simulink model "MBE_Simulation_04_Template_14_11_final"  (R2017b)
settings: Solver=FixedStepAuto  StartTime=0.0  StopTime=inf  FixedStep=0.05  RelTol=1e-3
libraries: simulink x67, canmsglib x4, instrumentlib x2, realtime_pacer_lib x1, hdlsllib x1
(part 1 of 4)
settings Model: Creator=holtv  LastModifiedBy=labadmin
settings CodeAppCC: StateflowObjectComments=on

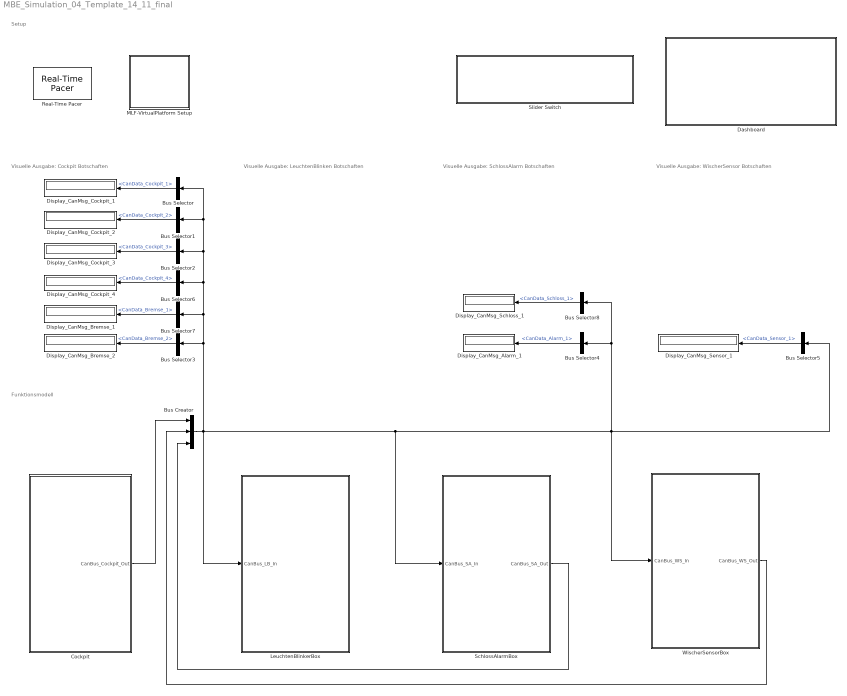
== system MBE_Simulation_04_Template_14_11_final ==
  note: Setup
  note: Visuelle Ausgabe: Cockpit Botschaften
  note: Funktionsmodell
  note: Visuelle Ausgabe: SchlossAlarm Botschaften
  note: Visuelle Ausgabe: LeuchtenBlinken Botschaften
  note: Visuelle Ausgabe: WischerSensor Botschaften
  Bus Creator : BusCreator  Inputs=3
  Bus Selector : BusSelector  OutputSignals=CanBus_Cockpit.CanMsg_Cockpit_1.CanData_Cockpit_1
  Bus Selector1 : BusSelector  OutputSignals=CanBus_Cockpit.CanMsg_Cockpit_2.CanData_Cockpit_2
  Bus Selector2 : BusSelector  OutputSignals=CanBus_Cockpit.CanMsg_Cockpit_3.CanData_Cockpit_3
  Bus Selector3 : BusSelector  OutputSignals=CanBus_Cockpit.CanMsg_Bremse_2.CanData_Bremse_2
  Bus Selector4 : BusSelector  OutputSignals=CanBus_SA.CanMsg_Alarm_1.CanData_Alarm_1
  Bus Selector5 : BusSelector  OutputSignals=CanBus_WS.CanMsg_Sensor_1.CanData_Sensor_1
  Bus Selector6 : BusSelector  OutputSignals=CanBus_Cockpit.CanMsg_Cockpit_4.CanData_Cockpit_4
  Bus Selector7 : BusSelector  OutputSignals=CanBus_Cockpit.CanMsg_Bremse_1.CanData_Bremse_1
  Bus Selector8 : BusSelector  OutputSignals=CanBus_SA.CanMsg_Schloss_1.CanData_Schloss_1
  Cockpit : Subsystem
  Dashboard : Subsystem
      mask Display: image('resources/simulink-dashboard.png');
  Display_CanMsg_Alarm_1 : Display
      settings: Format=binary (Stored Integer)
  Display_CanMsg_Bremse_1 : Display
      settings: Format=binary (Stored Integer)
  Display_CanMsg_Bremse_2 : Display
      settings: Format=binary (Stored Integer)
  Display_CanMsg_Cockpit_{1..4} (4 alike) : Display
      settings: Format=binary (Stored Integer)
  Display_CanMsg_Schloss_1 : Display
      settings: Format=binary (Stored Integer)
  Display_CanMsg_Sensor_1 : Display
      settings: Format=binary (Stored Integer)
  LeuchtenBlinkerBox : Subsystem
  MLF-VirtualPlatform Setup : Subsystem
  Real-Time Pacer : realtime_pacer_lib/Real-Time Pacer  simTimePerRealTime=1
  SchlossAlarmBox : Subsystem
  Slider Switch : Subsystem  DialogController=hmiCreateDDGDialog  IsWebBlock=on  mask(MWDashboardBlock){webBlockId=66e1d68e-5f4b-49dc-992d-d286b9288448, webBlockType=sliderswitch, ShowInLibBrowser=on, ShowInitialText=on, HMISrcModelName=MBE_Simulation_04_Template_14_11_final}
      mask prompts: webBlockId "WebBlock Id"; webBlockType "WebBlock Type"; HMISrcModelName "Source Model"
      mask help: Set on/off value to tune parameters or variables.
      mask Help: helpview([docroot '/mapfiles/simulink.map'], 'hmi_switch')
      mask Display:
      | if strcmp(get_param(bdroot(gcb),'BlockDiagramType'),'library')
      |  image([(matlabroot) '/toolbox/simulink/hmi/icons/SliderSwitch.png'])
      | end
  WischerSensorBox : Subsystem
  wires:
  Bus Creator/1 -> Bus Selector/1, Bus Selector1/1, Bus Selector2/1, Bus Selector6/1, Bus Selector7/1, Bus Selector3/1, Bus Selector5/1, Bus Selector8/1, Bus Selector4/1, WischerSensorBox/1(CanBus_WS_In), SchlossAlarmBox/1(CanBus_SA_In), LeuchtenBlinkerBox/1(CanBus_LB_In)
  Bus Selector/1 -> Display_CanMsg_Cockpit_1/1  "<CanData_Cockpit_1>"
  Bus Selector1/1 -> Display_CanMsg_Cockpit_2/1  "<CanData_Cockpit_2>"
  Bus Selector2/1 -> Display_CanMsg_Cockpit_3/1  "<CanData_Cockpit_3>"
  Bus Selector3/1 -> Display_CanMsg_Bremse_2/1  "<CanData_Bremse_2>"
  Bus Selector4/1 -> Display_CanMsg_Alarm_1/1  "<CanData_Alarm_1>"
  Bus Selector5/1 -> Display_CanMsg_Sensor_1/1  "<CanData_Sensor_1>"
  Cockpit/1(CanBus_Cockpit_Out) -> Bus Creator/1
  Bus Selector6/1 -> Display_CanMsg_Cockpit_4/1  "<CanData_Cockpit_4>"
  Bus Selector7/1 -> Display_CanMsg_Bremse_1/1  "<CanData_Bremse_1>"
  Bus Selector8/1 -> Display_CanMsg_Schloss_1/1  "<CanData_Schloss_1>"
  SchlossAlarmBox/1(CanBus_SA_Out) -> Bus Creator/3
  WischerSensorBox/1(CanBus_WS_Out) -> Bus Creator/2

== system MBE_Simulation_04_Template_14_11_final/Cockpit ==
  note: Applikation
  note: Simulation
  CanBus_Cockpit : Subsystem
  CanCoder_Bremse_1 : Subsystem
  CanCoder_Bremse_2 : Subsystem
  CanCoder_Cockpit_1 : Subsystem
  CanCoder_Cockpit_2 : Subsystem
  CanCoder_Cockpit_3 : Subsystem
  CanCoder_Cockpit_4 : Subsystem
  CanTransmit_Bremse_1 : Subsystem
  CanTransmit_Bremse_2 : Subsystem
  CanTransmit_Cockpit_1 : Subsystem
  CanTransmit_Cockpit_2 : Subsystem
  CanTransmit_Cockpit_3 : Subsystem
  CanTransmit_Cockpit_4 : Subsystem
  PanelInput_Cockpit : Subsystem
  CanBus_Cockpit_Out : Outport
  wires:
  PanelInput_Cockpit/1(LichtSwitch_Out) -> CanCoder_Cockpit_1/1(Lichtschalter_In)
  PanelInput_Cockpit/2(BlinkerSwitch_Out) -> CanCoder_Cockpit_1/2(Blinkerhebel_In)
  PanelInput_Cockpit/3(WarnblinkerSwitch_Out) -> CanCoder_Cockpit_1/3(Warnblinker)
  PanelInput_Cockpit/4(WischerSwitch_Out) -> CanCoder_Cockpit_2/1(WischerSwitch_In)
  PanelInput_Cockpit/5(WischWaschButton_Out) -> CanCoder_Cockpit_2/2(WischWaschButton_In)
  PanelInput_Cockpit/6(ScheibenheizungSwitch_Out) -> CanCoder_Cockpit_2/3(ScheibenheizungSwitch_In)
  PanelInput_Cockpit/7(TemperaturSlider_Out) -> CanCoder_Cockpit_2/4(TemperaturSlider_In)
  PanelInput_Cockpit/8(AlarmResetButton_Out) -> CanCoder_Cockpit_3/1(AlarmResetButton_In)
  PanelInput_Cockpit/13(GeschwindigkeitsSlider_Out) -> CanCoder_Bremse_2/1(GeschwindigkeitsSlider_In)
  PanelInput_Cockpit/9(IgnitionSwitch_Out) -> CanCoder_Cockpit_4/1(IgnitionSwitch_In)
  PanelInput_Cockpit/10(BremseButton_Out) -> CanCoder_Bremse_1/1(Bremse_In)
  PanelInput_Cockpit/11(WarnbremsungButton_Out) -> CanCoder_Bremse_1/2(Warnbremsung_In)
  PanelInput_Cockpit/12(NotbremsungButton_Out) -> CanCoder_Bremse_1/3(Notbremsungl_In)
  CanCoder_Cockpit_1/1(CanData_Cockpit_1) -> CanTransmit_Cockpit_1/1(CanData_Cockpit_1_In)  "CanData_Cockpit_1"
  CanCoder_Cockpit_1/2(CanTrigger_Cockpit_1) -> CanTransmit_Cockpit_1/2(CanTrigger_Cockpit_1_In)  "CanTrigger_Cockpit_1"
  CanCoder_Cockpit_2/1(CanData_Cockpit_2) -> CanTransmit_Cockpit_2/1(CanData_Cockpit_2_In)  "CanData_Cockpit_2"
  CanCoder_Cockpit_2/2(CanTrigger_Cockpit_2) -> CanTransmit_Cockpit_2/2(CanTrigger_Cockpit_2_In)  "CanTrigger_Cockpit_2"
  CanCoder_Cockpit_3/1(CanData_Cockpit_3) -> CanTransmit_Cockpit_3/1(CanData_Cockpit_3_In)  "CanData_Cockpit_3"
  CanCoder_Cockpit_3/2(CanTrigger_Cockpit_3) -> CanTransmit_Cockpit_3/2(CanTrigger_Cockpit_3_In)  "CanTrigger_Cockpit_3"
  CanCoder_Cockpit_4/1(CanData_Cockpit_4) -> CanTransmit_Cockpit_4/1(CanData_Cockpit_4_In)  "CanData_Cockpit_4"
  CanCoder_Cockpit_4/2(CanTrigger_Cockpit_4) -> CanTransmit_Cockpit_4/2(CanTrigger_Cockpit_4_In)  "CanTrigger_Cockpit_4"
  CanCoder_Bremse_1/1(CanData_Bremse_1) -> CanTransmit_Bremse_1/1(CanData_Bremse_1_In)  "CanData_Bremse_1"
  CanCoder_Bremse_1/2(CanTrigger_Bremse_1) -> CanTransmit_Bremse_1/2(CanTrigger_Bremse_1_In)  "CanTrigger_Bremse_1"
  CanCoder_Bremse_2/1(CanMsg_Bremse_2) -> CanTransmit_Bremse_2/1(CanData_Bremse_2_In)  "CanData_Bremse_2"
  CanCoder_Bremse_2/2(CanTrigger_Bremse_2) -> CanTransmit_Bremse_2/2(CanTrigger_Bremse_2_In)  "CanTrigger_Bremse_2"
  CanTransmit_Cockpit_1/1(CanMsg_Cockpit_1_Out) -> CanBus_Cockpit/1("CanMsg_Cockpit_1_In ")  "CanMsg_Cockpit_1"
  CanTransmit_Cockpit_2/1(CanMsg_Cockpit_2_Out) -> CanBus_Cockpit/2(CanMsg_Cockpit_2_In)  "CanMsg_Cockpit_2"
  CanTransmit_Cockpit_3/1(CanMsg_Cockpit_3_Out) -> CanBus_Cockpit/3(CanMsg_Cockpit_3_In)  "CanMsg_Cockpit_3"
  CanTransmit_Cockpit_4/1(CanMsg_Cockpit_4_Out) -> CanBus_Cockpit/4(CanMsg_Cockpit_4_In)  "CanMsg_Cockpit_4"
  CanTransmit_Bremse_1/1(CanTrigger_Bremse_1_Out) -> CanBus_Cockpit/5(CanMsg_Bremse_1_In)  "CanMsg_Bremse_1"
  CanTransmit_Bremse_2/1(CanMsg_Bremse_2_Out) -> CanBus_Cockpit/6(CanMsg_Bremse_2_In)  "CanMsg_Bremse_2"
  CanBus_Cockpit/1(CanBus_Cockpit_Out) -> CanBus_Cockpit_Out/1  "CanBus_Cockpit"

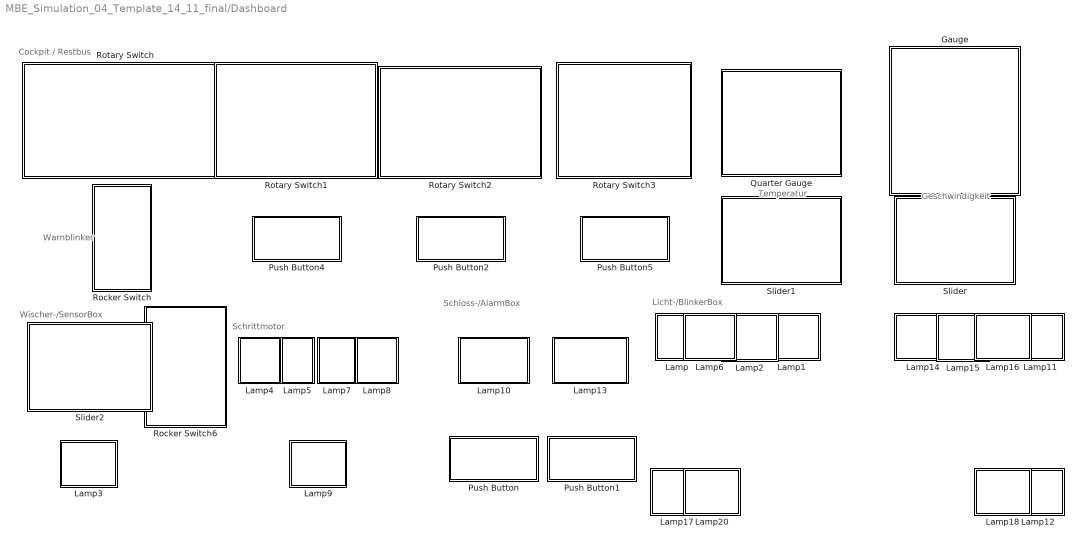
== system MBE_Simulation_04_Template_14_11_final/Dashboard ==
  note: Temperatur
  note: Geschwindigkeit
  note: Warnblinker
  note: Schloss-/AlarmBox
  note: Schrittmotor
  note: Wischer-/SensorBox
  note: Cockpit / Restbus
  note: Licht-/BlinkerBox
  Gauge : Subsystem  DialogController=hmiCreateDDGDialog  IsWebBlock=on  mask(MWDashboardBlock){webBlockId=ca009e5b-bc53-4e09-90f4-318b3a316375, webBlockType=circulargauge, ShowInLibBrowser=on, ShowInitialText=on, HMISrcModelName=MBE_Simulation_04_Template_14_11_final}
      mask prompts: webBlockId "WebBlock Id"; webBlockType "WebBlock Type"; HMISrcModelName "Source Model"
      mask help: Display an input value on a circular scale.
      mask Help: helpview([docroot '/mapfiles/simulink.map'], 'hmi_gauge')
      mask Display:
      | if strcmp(get_param(bdroot(gcb),'BlockDiagramType'),'library')
      |  image([(matlabroot) '/toolbox/simulink/hmi/icons/CircularGauge.png'])
      | end
  Lamp : Subsystem  DialogController=hmiCreateDDGDialog  IsWebBlock=on  mask(MWDashboardBlock){webBlockId=81971842-9de1-4b0d-b60d-6b7e37ec8366, webBlockType=lamp, ShowInLibBrowser=on, ShowInitialText=on, HMISrcModelName=MBE_Simulation_04_Template_14_11_final}
      mask prompts: webBlockId "WebBlock Id"; webBlockType "WebBlock Type"; HMISrcModelName "Source Model"
      mask help: Display a color that reflects an input value.
      mask Help: helpview([docroot '/mapfiles/simulink.map'], 'hmi_lamp')
      mask Display:
      | if strcmp(get_param(bdroot(gcb),'BlockDiagramType'),'library')
      |  image([(matlabroot) '/toolbox/simulink/hmi/icons/Lamp.png'])
      | end
  Lamp1 : Subsystem  DialogController=hmiCreateDDGDialog  IsWebBlock=on  mask(MWDashboardBlock){webBlockId=6164437f-0de0-4420-8afe-83f9f405fa61, webBlockType=lamp, ShowInLibBrowser=on, ShowInitialText=on, HMISrcModelName=MBE_Simulation_04_Template_14_11_final}
      mask prompts: webBlockId "WebBlock Id"; webBlockType "WebBlock Type"; HMISrcModelName "Source Model"
      mask help: Display a color that reflects an input value.
      mask Help: helpview([docroot '/mapfiles/simulink.map'], 'hmi_lamp')
      mask Display:
      | if strcmp(get_param(bdroot(gcb),'BlockDiagramType'),'library')
      |  image([(matlabroot) '/toolbox/simulink/hmi/icons/Lamp.png'])
      | end
  Lamp10 : Subsystem  DialogController=hmiCreateDDGDialog  IsWebBlock=on  mask(MWDashboardBlock){webBlockId=e0d27a18-3c75-41e4-afb0-c184a806c7c9, webBlockType=lamp, ShowInLibBrowser=on, ShowInitialText=on, HMISrcModelName=MBE_Simulation_04_Template_14_11_final}
      mask prompts: webBlockId "WebBlock Id"; webBlockType "WebBlock Type"; HMISrcModelName "Source Model"
      mask help: Display a color that reflects an input value.
      mask Help: helpview([docroot '/mapfiles/simulink.map'], 'hmi_lamp')
      mask Display:
      | if strcmp(get_param(bdroot(gcb),'BlockDiagramType'),'library')
      |  image([(matlabroot) '/toolbox/simulink/hmi/icons/Lamp.png'])
      | end
  Lamp11 : Subsystem  DialogController=hmiCreateDDGDialog  IsWebBlock=on  mask(MWDashboardBlock){webBlockId=03ea03de-7c81-41a7-863d-ac3bb75d845f, webBlockType=lamp, ShowInLibBrowser=on, ShowInitialText=on, HMISrcModelName=MBE_Simulation_04_Template_14_11_final}
      mask prompts: webBlockId "WebBlock Id"; webBlockType "WebBlock Type"; HMISrcModelName "Source Model"
      mask help: Display a color that reflects an input value.
      mask Help: helpview([docroot '/mapfiles/simulink.map'], 'hmi_lamp')
      mask Display:
      | if strcmp(get_param(bdroot(gcb),'BlockDiagramType'),'library')
      |  image([(matlabroot) '/toolbox/simulink/hmi/icons/Lamp.png'])
      | end
  Lamp12 : Subsystem  DialogController=hmiCreateDDGDialog  IsWebBlock=on  mask(MWDashboardBlock){webBlockId=0e17ce2a-30cc-4796-9e12-573dab1135c9, webBlockType=lamp, ShowInLibBrowser=on, ShowInitialText=on, HMISrcModelName=MBE_Simulation_04_Template_14_11_final}
      mask prompts: webBlockId "WebBlock Id"; webBlockType "WebBlock Type"; HMISrcModelName "Source Model"
      mask help: Display a color that reflects an input value.
      mask Help: helpview([docroot '/mapfiles/simulink.map'], 'hmi_lamp')
      mask Display:
      | if strcmp(get_param(bdroot(gcb),'BlockDiagramType'),'library')
      |  image([(matlabroot) '/toolbox/simulink/hmi/icons/Lamp.png'])
      | end
  Lamp13 : Subsystem  DialogController=hmiCreateDDGDialog  IsWebBlock=on  mask(MWDashboardBlock){webBlockId=2f548181-9e42-4df5-9bf9-2368ca2048ef, webBlockType=lamp, ShowInLibBrowser=on, ShowInitialText=on, HMISrcModelName=MBE_Simulation_04_Template_14_11_final}
      mask prompts: webBlockId "WebBlock Id"; webBlockType "WebBlock Type"; HMISrcModelName "Source Model"
      mask help: Display a color that reflects an input value.
      mask Help: helpview([docroot '/mapfiles/simulink.map'], 'hmi_lamp')
      mask Display:
      | if strcmp(get_param(bdroot(gcb),'BlockDiagramType'),'library')
      |  image([(matlabroot) '/toolbox/simulink/hmi/icons/Lamp.png'])
      | end
  Lamp14 : Subsystem  DialogController=hmiCreateDDGDialog  IsWebBlock=on  mask(MWDashboardBlock){webBlockId=695a449a-89c0-4648-941b-7901b844a223, webBlockType=lamp, ShowInLibBrowser=on, ShowInitialText=on, HMISrcModelName=MBE_Simulation_04_Template_14_11_final}
      mask prompts: webBlockId "WebBlock Id"; webBlockType "WebBlock Type"; HMISrcModelName "Source Model"
      mask help: Display a color that reflects an input value.
      mask Help: helpview([docroot '/mapfiles/simulink.map'], 'hmi_lamp')
      mask Display:
      | if strcmp(get_param(bdroot(gcb),'BlockDiagramType'),'library')
      |  image([(matlabroot) '/toolbox/simulink/hmi/icons/Lamp.png'])
      | end
  Lamp15 : Subsystem  DialogController=hmiCreateDDGDialog  IsWebBlock=on  mask(MWDashboardBlock){webBlockId=ab847f27-61fc-4651-8680-973b52bd2ee5, webBlockType=lamp, ShowInLibBrowser=on, ShowInitialText=on, HMISrcModelName=MBE_Simulation_04_Template_14_11_final}
      mask prompts: webBlockId "WebBlock Id"; webBlockType "WebBlock Type"; HMISrcModelName "Source Model"
      mask help: Display a color that reflects an input value.
      mask Help: helpview([docroot '/mapfiles/simulink.map'], 'hmi_lamp')
      mask Display:
      | if strcmp(get_param(bdroot(gcb),'BlockDiagramType'),'library')
      |  image([(matlabroot) '/toolbox/simulink/hmi/icons/Lamp.png'])
      | end
  Lamp16 : Subsystem  DialogController=hmiCreateDDGDialog  IsWebBlock=on  mask(MWDashboardBlock){webBlockId=4b59acee-b734-4497-ab44-301c6843ab2b, webBlockType=lamp, ShowInLibBrowser=on, ShowInitialText=on, HMISrcModelName=MBE_Simulation_04_Template_14_11_final}
      mask prompts: webBlockId "WebBlock Id"; webBlockType "WebBlock Type"; HMISrcModelName "Source Model"
      mask help: Display a color that reflects an input value.
      mask Help: helpview([docroot '/mapfiles/simulink.map'], 'hmi_lamp')
      mask Display:
      | if strcmp(get_param(bdroot(gcb),'BlockDiagramType'),'library')
      |  image([(matlabroot) '/toolbox/simulink/hmi/icons/Lamp.png'])
      | end
  Lamp17 : Subsystem  DialogController=hmiCreateDDGDialog  IsWebBlock=on  mask(MWDashboardBlock){webBlockId=786eefba-2348-4559-8fc8-a6cc7c921991, webBlockType=lamp, ShowInLibBrowser=on, ShowInitialText=on, HMISrcModelName=MBE_Simulation_04_Template_14_11_final}
      mask prompts: webBlockId "WebBlock Id"; webBlockType "WebBlock Type"; HMISrcModelName "Source Model"
      mask help: Display a color that reflects an input value.
      mask Help: helpview([docroot '/mapfiles/simulink.map'], 'hmi_lamp')
      mask Display:
      | if strcmp(get_param(bdroot(gcb),'BlockDiagramType'),'library')
      |  image([(matlabroot) '/toolbox/simulink/hmi/icons/Lamp.png'])
      | end
  Lamp18 : Subsystem  DialogController=hmiCreateDDGDialog  IsWebBlock=on  mask(MWDashboardBlock){webBlockId=1ccec556-46b1-4b1b-9c3b-62947f75bff4, webBlockType=lamp, ShowInLibBrowser=on, ShowInitialText=on, HMISrcModelName=MBE_Simulation_04_Template_14_11_final}
      mask prompts: webBlockId "WebBlock Id"; webBlockType "WebBlock Type"; HMISrcModelName "Source Model"
      mask help: Display a color that reflects an input value.
      mask Help: helpview([docroot '/mapfiles/simulink.map'], 'hmi_lamp')
      mask Display:
      | if strcmp(get_param(bdroot(gcb),'BlockDiagramType'),'library')
      |  image([(matlabroot) '/toolbox/simulink/hmi/icons/Lamp.png'])
      | end
  Lamp2 : Subsystem  DialogController=hmiCreateDDGDialog  IsWebBlock=on  mask(MWDashboardBlock){webBlockId=47b8fd33-47ee-48e2-8eae-e8ebe4084eb8, webBlockType=lamp, ShowInLibBrowser=on, ShowInitialText=on, HMISrcModelName=MBE_Simulation_04_Template_14_11_final}
      mask prompts: webBlockId "WebBlock Id"; webBlockType "WebBlock Type"; HMISrcModelName "Source Model"
      mask help: Display a color that reflects an input value.
      mask Help: helpview([docroot '/mapfiles/simulink.map'], 'hmi_lamp')
      mask Display:
      | if strcmp(get_param(bdroot(gcb),'BlockDiagramType'),'library')
      |  image([(matlabroot) '/toolbox/simulink/hmi/icons/Lamp.png'])
      | end
  Lamp20 : Subsystem  DialogController=hmiCreateDDGDialog  IsWebBlock=on  mask(MWDashboardBlock){webBlockId=931f0f15-782b-4b6b-a159-35edc5b1fde3, webBlockType=lamp, ShowInLibBrowser=on, ShowInitialText=on, HMISrcModelName=MBE_Simulation_04_Template_14_11_final}
      mask prompts: webBlockId "WebBlock Id"; webBlockType "WebBlock Type"; HMISrcModelName "Source Model"
      mask help: Display a color that reflects an input value.
      mask Help: helpview([docroot '/mapfiles/simulink.map'], 'hmi_lamp')
      mask Display:
      | if strcmp(get_param(bdroot(gcb),'BlockDiagramType'),'library')
      |  image([(matlabroot) '/toolbox/simulink/hmi/icons/Lamp.png'])
      | end
  Lamp3 : Subsystem  DialogController=hmiCreateDDGDialog  IsWebBlock=on  mask(MWDashboardBlock){webBlockId=dd43efa0-be9c-4aa7-8a6b-057b24033f5b, webBlockType=lamp, ShowInLibBrowser=on, ShowInitialText=on, HMISrcModelName=MBE_Simulation_04_Template_14_11_final}
      mask prompts: webBlockId "WebBlock Id"; webBlockType "WebBlock Type"; HMISrcModelName "Source Model"
      mask help: Display a color that reflects an input value.
      mask Help: helpview([docroot '/mapfiles/simulink.map'], 'hmi_lamp')
      mask Display:
      | if strcmp(get_param(bdroot(gcb),'BlockDiagramType'),'library')
      |  image([(matlabroot) '/toolbox/simulink/hmi/icons/Lamp.png'])
      | end
  Lamp4 : Subsystem  DialogController=hmiCreateDDGDialog  IsWebBlock=on  mask(MWDashboardBlock){webBlockId=ec470312-b7a9-47e7-bff1-3dfc60bd552b, webBlockType=lamp, ShowInLibBrowser=on, ShowInitialText=on, HMISrcModelName=MBE_Simulation_04_Template_14_11_final}
      mask prompts: webBlockId "WebBlock Id"; webBlockType "WebBlock Type"; HMISrcModelName "Source Model"
      mask help: Display a color that reflects an input value.
      mask Help: helpview([docroot '/mapfiles/simulink.map'], 'hmi_lamp')
      mask Display:
      | if strcmp(get_param(bdroot(gcb),'BlockDiagramType'),'library')
      |  image([(matlabroot) '/toolbox/simulink/hmi/icons/Lamp.png'])
      | end
  Lamp5 : Subsystem  DialogController=hmiCreateDDGDialog  IsWebBlock=on  mask(MWDashboardBlock){webBlockId=c417e66f-c67a-45c5-93e6-a2e61e7ee47f, webBlockType=lamp, ShowInLibBrowser=on, ShowInitialText=on, HMISrcModelName=MBE_Simulation_04_Template_14_11_final}
      mask prompts: webBlockId "WebBlock Id"; webBlockType "WebBlock Type"; HMISrcModelName "Source Model"
      mask help: Display a color that reflects an input value.
      mask Help: helpview([docroot '/mapfiles/simulink.map'], 'hmi_lamp')
      mask Display:
      | if strcmp(get_param(bdroot(gcb),'BlockDiagramType'),'library')
      |  image([(matlabroot) '/toolbox/simulink/hmi/icons/Lamp.png'])
      | end
  Lamp6 : Subsystem  DialogController=hmiCreateDDGDialog  IsWebBlock=on  mask(MWDashboardBlock){webBlockId=25372d07-c1b6-4919-ab6c-b02a672d7981, webBlockType=lamp, ShowInLibBrowser=on, ShowInitialText=on, HMISrcModelName=MBE_Simulation_04_Template_14_11_final}
      mask prompts: webBlockId "WebBlock Id"; webBlockType "WebBlock Type"; HMISrcModelName "Source Model"
      mask help: Display a color that reflects an input value.
      mask Help: helpview([docroot '/mapfiles/simulink.map'], 'hmi_lamp')
      mask Display:
      | if strcmp(get_param(bdroot(gcb),'BlockDiagramType'),'library')
      |  image([(matlabroot) '/toolbox/simulink/hmi/icons/Lamp.png'])
      | end
  Lamp7 : Subsystem  DialogController=hmiCreateDDGDialog  IsWebBlock=on  mask(MWDashboardBlock){webBlockId=453b9024-6720-4083-84ad-643553e1bf92, webBlockType=lamp, ShowInLibBrowser=on, ShowInitialText=on, HMISrcModelName=MBE_Simulation_04_Template_14_11_final}
      mask prompts: webBlockId "WebBlock Id"; webBlockType "WebBlock Type"; HMISrcModelName "Source Model"
      mask help: Display a color that reflects an input value.
      mask Help: helpview([docroot '/mapfiles/simulink.map'], 'hmi_lamp')
      mask Display:
      | if strcmp(get_param(bdroot(gcb),'BlockDiagramType'),'library')
      |  image([(matlabroot) '/toolbox/simulink/hmi/icons/Lamp.png'])
      | end
  Lamp8 : Subsystem  DialogController=hmiCreateDDGDialog  IsWebBlock=on  mask(MWDashboardBlock){webBlockId=65a73d86-464d-4cc4-bc4b-89bd3b5f1893, webBlockType=lamp, ShowInLibBrowser=on, ShowInitialText=on, HMISrcModelName=MBE_Simulation_04_Template_14_11_final}
      mask prompts: webBlockId "WebBlock Id"; webBlockType "WebBlock Type"; HMISrcModelName "Source Model"
      mask help: Display a color that reflects an input value.
      mask Help: helpview([docroot '/mapfiles/simulink.map'], 'hmi_lamp')
      mask Display:
      | if strcmp(get_param(bdroot(gcb),'BlockDiagramType'),'library')
      |  image([(matlabroot) '/toolbox/simulink/hmi/icons/Lamp.png'])
      | end
  Lamp9 : Subsystem  DialogController=hmiCreateDDGDialog  IsWebBlock=on  mask(MWDashboardBlock){webBlockId=1c7a1f23-4597-47ed-8943-470ce80c9288, webBlockType=lamp, ShowInLibBrowser=on, ShowInitialText=on, HMISrcModelName=MBE_Simulation_04_Template_14_11_final}
      mask prompts: webBlockId "WebBlock Id"; webBlockType "WebBlock Type"; HMISrcModelName "Source Model"
      mask help: Display a color that reflects an input value.
      mask Help: helpview([docroot '/mapfiles/simulink.map'], 'hmi_lamp')
      mask Display:
      | if strcmp(get_param(bdroot(gcb),'BlockDiagramType'),'library')
      |  image([(matlabroot) '/toolbox/simulink/hmi/icons/Lamp.png'])
      | end
  Push Button : Subsystem  DialogController=hmiCreateDDGDialog  IsWebBlock=on  mask(MWDashboardBlock){webBlockId=62e63348-a91a-44a9-b1e9-60eeb391ed6f, webBlockType=pushbutton, ShowInLibBrowser=on, ShowInitialText=on, HMISrcModelName=MBE_Simulation_04_Template_14_11_final}
      mask prompts: webBlockId "WebBlock Id"; webBlockType "WebBlock Type"; HMISrcModelName "Source Model"
      mask help: Set a value of a tunable parameter or variable by holding the button. When you release the button, the value of the connected parameter or variable is set back to the default.
      mask Help: helpview([docroot '/mapfiles/simulink.map'], 'hmi_pushbutton')
      mask Display:
      | if strcmp(get_param(bdroot(gcb),'BlockDiagramType'),'library')
      |  image([(matlabroot) '/toolbox/simulink/hmi/icons/PushButton.png'])
      | end
  Push Button1 : Subsystem  DialogController=hmiCreateDDGDialog  IsWebBlock=on  mask(MWDashboardBlock){webBlockId=ca334dcf-1f9e-4867-b238-ceadcdcd4037, webBlockType=pushbutton, ShowInLibBrowser=on, ShowInitialText=on, HMISrcModelName=MBE_Simulation_04_Template_14_11_final}
      mask prompts: webBlockId "WebBlock Id"; webBlockType "WebBlock Type"; HMISrcModelName "Source Model"
      mask help: Set a value of a tunable parameter or variable by holding the button. When you release the button, the value of the connected parameter or variable is set back to the default.
      mask Help: helpview([docroot '/mapfiles/simulink.map'], 'hmi_pushbutton')
      mask Display:
      | if strcmp(get_param(bdroot(gcb),'BlockDiagramType'),'library')
      |  image([(matlabroot) '/toolbox/simulink/hmi/icons/PushButton.png'])
      | end
  Push Button2 : Subsystem  DialogController=hmiCreateDDGDialog  IsWebBlock=on  mask(MWDashboardBlock){webBlockId=e9f72392-2ca9-46af-ad7d-d12fc7ba9ad6, webBlockType=pushbutton, ShowInLibBrowser=on, ShowInitialText=on, HMISrcModelName=MBE_Simulation_04_Template_14_11_final}
      mask prompts: webBlockId "WebBlock Id"; webBlockType "WebBlock Type"; HMISrcModelName "Source Model"
      mask help: Set a value of a tunable parameter or variable by holding the button. When you release the button, the value of the connected parameter or variable is set back to the default.
      mask Help: helpview([docroot '/mapfiles/simulink.map'], 'hmi_pushbutton')
      mask Display:
      | if strcmp(get_param(bdroot(gcb),'BlockDiagramType'),'library')
      |  image([(matlabroot) '/toolbox/simulink/hmi/icons/PushButton.png'])
      | end
  Push Button4 : Subsystem  DialogController=hmiCreateDDGDialog  IsWebBlock=on  mask(MWDashboardBlock){webBlockId=5a2cf449-0cca-4fb7-b784-159269e12d6e, webBlockType=pushbutton, ShowInLibBrowser=on, ShowInitialText=on, HMISrcModelName=MBE_Simulation_04_Template_14_11_final}
      mask prompts: webBlockId "WebBlock Id"; webBlockType "WebBlock Type"; HMISrcModelName "Source Model"
      mask help: Set a value of a tunable parameter or variable by holding the button. When you release the button, the value of the connected parameter or variable is set back to the default.
      mask Help: helpview([docroot '/mapfiles/simulink.map'], 'hmi_pushbutton')
      mask Display:
      | if strcmp(get_param(bdroot(gcb),'BlockDiagramType'),'library')
      |  image([(matlabroot) '/toolbox/simulink/hmi/icons/PushButton.png'])
      | end
  Push Button5 : Subsystem  DialogController=hmiCreateDDGDialog  IsWebBlock=on  mask(MWDashboardBlock){webBlockId=5c67a276-91f8-4d4c-bcd3-2351cc1ea837, webBlockType=pushbutton, ShowInLibBrowser=on, ShowInitialText=on, HMISrcModelName=MBE_Simulation_04_Template_14_11_final}
      mask prompts: webBlockId "WebBlock Id"; webBlockType "WebBlock Type"; HMISrcModelName "Source Model"
      mask help: Set a value of a tunable parameter or variable by holding the button. When you release the button, the value of the connected parameter or variable is set back to the default.
      mask Help: helpview([docroot '/mapfiles/simulink.map'], 'hmi_pushbutton')
      mask Display:
      | if strcmp(get_param(bdroot(gcb),'BlockDiagramType'),'library')
      |  image([(matlabroot) '/toolbox/simulink/hmi/icons/PushButton.png'])
      | end
  Quarter Gauge : Subsystem  DialogController=hmiCreateDDGDialog  IsWebBlock=on  mask(MWDashboardBlock){webBlockId=b5c302db-c61a-421c-8a53-531e84cf8cf2, webBlockType=ninetydegreegauge, ShowInLibBrowser=on, ShowInitialText=on, HMISrcModelName=MBE_Simulation_04_Template_14_11_final}
      mask prompts: webBlockId "WebBlock Id"; webBlockType "WebBlock Type"; HMISrcModelName "Source Model"
      mask help: Display an input value on a ninety degree scale.
      mask Help: helpview([docroot '/mapfiles/simulink.map'], 'hmi_quarter_gauge')
      mask Display:
      | if strcmp(get_param(bdroot(gcb),'BlockDiagramType'),'library')
      |  image([(matlabroot) '/toolbox/simulink/hmi/icons/NinetyDegreeGauge.png'])
      | end
  Rocker Switch : Subsystem  DialogController=hmiCreateDDGDialog  IsWebBlock=on  mask(MWDashboardBlock){webBlockId=3f04bdf2-d91a-4ceb-9013-8a892ff0acf2, webBlockType=rockerswitch, ShowInLibBrowser=on, ShowInitialText=on, HMISrcModelName=MBE_Simulation_04_Template_14_11_final}
      mask prompts: webBlockId "WebBlock Id"; webBlockType "WebBlock Type"; HMISrcModelName "Source Model"
      mask help: Set on/off value to tune parameters or variables.
      mask Help: helpview([docroot '/mapfiles/simulink.map'], 'hmi_switch')
      mask Display:
      | if strcmp(get_param(bdroot(gcb),'BlockDiagramType'),'library')
      |  image([(matlabroot) '/toolbox/simulink/hmi/icons/RockerSwitch.png'])
      | end
  Rocker Switch6 : Subsystem  DialogController=hmiCreateDDGDialog  IsWebBlock=on  mask(MWDashboardBlock){webBlockId=c047bee7-4707-46a7-a99a-ffd82d015350, webBlockType=rockerswitch, ShowInLibBrowser=on, ShowInitialText=on, HMISrcModelName=MBE_Simulation_04_Template_14_11_final}
      mask prompts: webBlockId "WebBlock Id"; webBlockType "WebBlock Type"; HMISrcModelName "Source Model"
      mask help: Set on/off value to tune parameters or variables.
      mask Help: helpview([docroot '/mapfiles/simulink.map'], 'hmi_switch')
      mask Display:
      | if strcmp(get_param(bdroot(gcb),'BlockDiagramType'),'library')
      |  image([(matlabroot) '/toolbox/simulink/hmi/icons/RockerSwitch.png'])
      | end
  Rotary Switch : Subsystem  DialogController=hmiCreateDDGDialog  IsWebBlock=on  mask(MWDashboardBlock){webBlockId=6d6f1039-d173-4f24-b8b6-fae1bd310954, webBlockType=discreteknob, ShowInLibBrowser=on, ShowInitialText=on, HMISrcModelName=MBE_Simulation_04_Template_14_11_final}
      mask prompts: webBlockId "WebBlock Id"; webBlockType "WebBlock Type"; HMISrcModelName "Source Model"
      mask help: Set value to tune parameters or variables.
      mask Help: helpview([docroot '/mapfiles/simulink.map'], 'hmi_rotary_switch')
      mask Display:
      | if strcmp(get_param(bdroot(gcb),'BlockDiagramType'),'library')
      |  image([(matlabroot) '/toolbox/simulink/hmi/icons/DiscreteKnob.png'])
      | end
  Rotary Switch1 : Subsystem  DialogController=hmiCreateDDGDialog  IsWebBlock=on  mask(MWDashboardBlock){webBlockId=65af94a3-58c4-401e-9577-5b6a4461a446, webBlockType=discreteknob, ShowInLibBrowser=on, ShowInitialText=on, HMISrcModelName=MBE_Simulation_04_Template_14_11_final}
      mask prompts: webBlockId "WebBlock Id"; webBlockType "WebBlock Type"; HMISrcModelName "Source Model"
      mask help: Set value to tune parameters or variables.
      mask Help: helpview([docroot '/mapfiles/simulink.map'], 'hmi_rotary_switch')
      mask Display:
      | if strcmp(get_param(bdroot(gcb),'BlockDiagramType'),'library')
      |  image([(matlabroot) '/toolbox/simulink/hmi/icons/DiscreteKnob.png'])
      | end
  Rotary Switch2 : Subsystem  DialogController=hmiCreateDDGDialog  IsWebBlock=on  mask(MWDashboardBlock){webBlockId=21516cb2-0aa3-42b1-834c-f92b883ef071, webBlockType=discreteknob, ShowInLibBrowser=on, ShowInitialText=on, HMISrcModelName=MBE_Simulation_04_Template_14_11_final}
      mask prompts: webBlockId "WebBlock Id"; webBlockType "WebBlock Type"; HMISrcModelName "Source Model"
      mask help: Set value to tune parameters or variables.
      mask Help: helpview([docroot '/mapfiles/simulink.map'], 'hmi_rotary_switch')
      mask Display:
      | if strcmp(get_param(bdroot(gcb),'BlockDiagramType'),'library')
      |  image([(matlabroot) '/toolbox/simulink/hmi/icons/DiscreteKnob.png'])
      | end
  Rotary Switch3 : Subsystem  DialogController=hmiCreateDDGDialog  IsWebBlock=on  mask(MWDashboardBlock){webBlockId=26fedd6e-6486-4e12-a782-e762a2dbf39d, webBlockType=discreteknob, ShowInLibBrowser=on, ShowInitialText=on, HMISrcModelName=MBE_Simulation_04_Template_14_11_final}
      mask prompts: webBlockId "WebBlock Id"; webBlockType "WebBlock Type"; HMISrcModelName "Source Model"
      mask help: Set value to tune parameters or variables.
      mask Help: helpview([docroot '/mapfiles/simulink.map'], 'hmi_rotary_switch')
      mask Display:
      | if strcmp(get_param(bdroot(gcb),'BlockDiagramType'),'library')
      |  image([(matlabroot) '/toolbox/simulink/hmi/icons/DiscreteKnob.png'])
      | end
  Slider : Subsystem  DialogController=hmiCreateDDGDialog  IsWebBlock=on  mask(MWDashboardBlock){webBlockId=764f1586-c564-476a-b65f-30263a131a1b, webBlockType=slider, ShowInLibBrowser=on, ShowInitialText=on, HMISrcModelName=MBE_Simulation_04_Template_14_11_final}
      mask prompts: webBlockId "WebBlock Id"; webBlockType "WebBlock Type"; HMISrcModelName "Source Model"
      mask help: Set value to tune parameters or variables.
      mask Help: helpview([docroot '/mapfiles/simulink.map'], 'hmi_slider')
      mask Display:
      | if strcmp(get_param(bdroot(gcb),'BlockDiagramType'),'library')
      |  image([(matlabroot) '/toolbox/simulink/hmi/icons/Slider.png'])
      | end
  Slider1 : Subsystem  DialogController=hmiCreateDDGDialog  IsWebBlock=on  mask(MWDashboardBlock){webBlockId=1d9575c2-d437-452f-9d8a-f62906f47bbe, webBlockType=slider, ShowInLibBrowser=on, ShowInitialText=on, HMISrcModelName=MBE_Simulation_04_Template_14_11_final}
      mask prompts: webBlockId "WebBlock Id"; webBlockType "WebBlock Type"; HMISrcModelName "Source Model"
      mask help: Set value to tune parameters or variables.
      mask Help: helpview([docroot '/mapfiles/simulink.map'], 'hmi_slider')
      mask Display:
      | if strcmp(get_param(bdroot(gcb),'BlockDiagramType'),'library')
      |  image([(matlabroot) '/toolbox/simulink/hmi/icons/Slider.png'])
      | end
  Slider2 : Subsystem  DialogController=hmiCreateDDGDialog  IsWebBlock=on  mask(MWDashboardBlock){webBlockId=ea16f3fa-bd80-460c-9323-1f43cc8cc32e, webBlockType=slider, ShowInLibBrowser=on, ShowInitialText=on, HMISrcModelName=MBE_Simulation_04_Template_14_11_final}
      mask prompts: webBlockId "WebBlock Id"; webBlockType "WebBlock Type"; HMISrcModelName "Source Model"
      mask help: Set value to tune parameters or variables.
      mask Help: helpview([docroot '/mapfiles/simulink.map'], 'hmi_slider')
      mask Display:
      | if strcmp(get_param(bdroot(gcb),'BlockDiagramType'),'library')
      |  image([(matlabroot) '/toolbox/simulink/hmi/icons/Slider.png'])
      | end

== system MBE_Simulation_04_Template_14_11_final/LeuchtenBlinkerBox ==
  CanBus_LB_In : Inport
  LB_Box_Applikation : Subsystem
  LB_Box_Simulation_Input : Subsystem
  LB_Box_Simulation_Output : Subsystem
  wires:
  CanBus_LB_In/1 -> LB_Box_Simulation_Input/1(CanBus_LB_In)
  LB_Box_Simulation_Input/2(CanData_Cockpit_1_Out) -> LB_Box_Applikation/2(CanData_Cockpit_1_In)
  LB_Box_Simulation_Input/3(CanTrigger_Cockpit_1_Out) -> LB_Box_Applikation/3(CanTrigger_Cockpit_1_In)
  LB_Box_Simulation_Input/4(CanData_Schloss_1_Out) -> LB_Box_Applikation/4(CanData_Schloss_1_In)
  LB_Box_Simulation_Input/5(CanTrigger_Schloss_1_Out) -> LB_Box_Applikation/5(CanTrigger_Schloss_1_In)
  LB_Box_Simulation_Input/6(CanData_Alarm_1_Out) -> LB_Box_Applikation/6(CanData_Alarm_1_In)
  LB_Box_Simulation_Input/7(CanTrigger_Alarm_1_Out) -> LB_Box_Applikation/7(CanTrigger_Alarm_1_In)
  LB_Box_Simulation_Input/8(CanData_Sensor_1_Out) -> LB_Box_Applikation/8(CanData_Sensor_1_In)
  LB_Box_Simulation_Input/9(CanTrigger_Sensor_1_Out) -> LB_Box_Applikation/9(CanTrigger_Sensor_1_In)
  LB_Box_Simulation_Input/10(CanData_Bremse_1_Out) -> LB_Box_Applikation/10(CanData_Bremse_1_In)
  LB_Box_Simulation_Input/11(CanTrigger_Bremse_1_Out) -> LB_Box_Applikation/11(CanTrigger_Bremse_1_In)
  LB_Box_Applikation/5(FEL_LED_Out) -> LB_Box_Simulation_Output/5(FEL_LED)
  LB_Box_Applikation/6(ABL_LED_Out) -> LB_Box_Simulation_Output/6(ABL_LED)
  LB_Box_Applikation/7(TFL_LED_Out) -> LB_Box_Simulation_Output/7(TFL_LED)
  LB_Box_Applikation/8(BLL_LED_Out) -> LB_Box_Simulation_Output/8(BLL_LED)
  LB_Box_Applikation/9(BLR_LED_Out) -> LB_Box_Simulation_Output/9(BLR_LED)
  LB_Box_Applikation/10(BRL_LED_Out) -> LB_Box_Simulation_Output/10(BRL_LED)
  LB_Box_Simulation_Input/1(GenericButton_Out) -> LB_Box_Applikation/1(GenericButton_In)
  LB_Box_Applikation/4(GenericLedOben_Out) -> LB_Box_Simulation_Output/4(GenericLedOben_LED_In)
  LB_Box_Applikation/3(GenericLedRechts_Out) -> LB_Box_Simulation_Output/3(GenericLedRechts_LED_In)
  LB_Box_Applikation/2(GenericLedLinks_Out) -> LB_Box_Simulation_Output/2(GenericLedLinks_LED_In)
  LB_Box_Applikation/1(GenericLedUnten_Out) -> LB_Box_Simulation_Output/1(GenericLedUnten_LED_In)
  LB_Box_Applikation/11(RL_LED_Out) -> LB_Box_Simulation_Output/11(RL_LED)
  LB_Box_Applikation/12(NSL_LED_Out) -> LB_Box_Simulation_Output/12(NSL_LED)
  LB_Box_Applikation/13(NSR_LED_Out) -> LB_Box_Simulation_Output/13(NSR_LED)
  LB_Box_Applikation/14(RFL_LED_Out) -> LB_Box_Simulation_Output/14(RFL_LED)

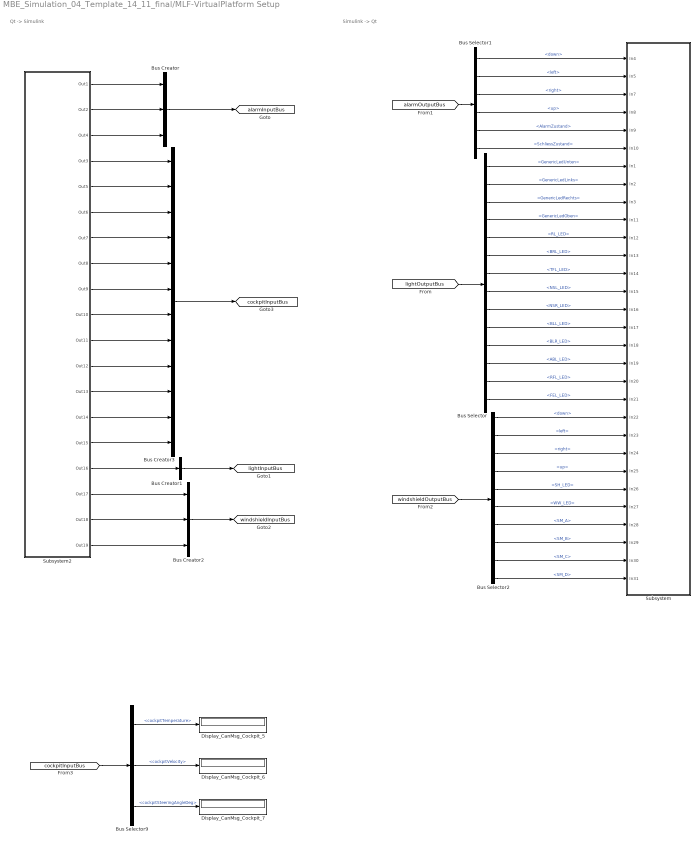
== system MBE_Simulation_04_Template_14_11_final/MLF-VirtualPlatform Setup ==
  note: Qt -> Simulink
  note: Simulink -> Qt
  Bus Creator : BusCreator  Inputs=3
  Bus Creator1 : BusCreator  Inputs=1
  Bus Creator2 : BusCreator  Inputs=3
  Bus Creator3 : BusCreator  Inputs=12
  Bus Selector : BusSelector  OutputSignals=GenericLedUnten,GenericLedLinks,GenericLedRechts,GenericLedOben,RL_LED,BRL_LED,TFL_LED,NSL_LED,NSR_LED,BLL_LED,BLR_LED,ABL_LED,RFL_LED,FEL_LED
  Bus Selector1 : BusSelector  OutputSignals=down,left,right,up,AlarmZustand,SchliessZustand
  Bus Selector2 : BusSelector  OutputSignals=down,left,right,up,SH_LED,WW_LED,SM_A,SM_B,SM_C,SM_D
  Bus Selector9 : BusSelector  OutputSignals=cockpitTemperature,cockpitVelocity,cockpitSteeringAngleDeg
  Display_CanMsg_Cockpit_5 : Display
      settings: Format=binary (Stored Integer)
  Display_CanMsg_Cockpit_6 : Display
      settings: Format=binary (Stored Integer)
  Display_CanMsg_Cockpit_7 : Display
      settings: Format=binary (Stored Integer)
  Subsystem : Subsystem
  Subsystem2 : Subsystem
  tag scope: alarmInputBus=global, cockpitInputBus=global, lightInputBus=global, windshieldInputBus=global
  wires:
  [lightOutputBus] -> Bus Selector/1
  Bus Selector/14 -> Subsystem/20(In21)  "<FEL_LED>"
  Bus Selector/12 -> Subsystem/18(In19)  "<ABL_LED>"
  Bus Selector/7 -> Subsystem/13(In14)  "<TFL_LED>"
  Bus Selector/10 -> Subsystem/16(In17)  "<BLL_LED>"
  Bus Selector/11 -> Subsystem/17(In18)  "<BLR_LED>"
  Bus Selector/1 -> Subsystem/7(In1)  "<GenericLedUnten>"
  [alarmOutputBus] -> Bus Selector1/1
  Subsystem2/3(Out4) -> Bus Creator/3
  Subsystem2/2(Out2) -> Bus Creator/2
  Subsystem2/1(Out1) -> Bus Creator/1
  Bus Creator/1 -> [alarmInputBus]
  Bus Selector1/5 -> Subsystem/5(In9)  "<AlarmZustand>"
  Bus Selector1/4 -> Subsystem/4(In8)  "<up>"
  Bus Selector1/3 -> Subsystem/3(In7)  "<right>"
  Bus Selector1/2 -> Subsystem/2(In5)  "<left>"
  Subsystem2/16(Out16) -> Bus Creator1/1
  Bus Creator1/1 -> [lightInputBus]
  Subsystem2/17(Out17) -> Bus Creator2/1
  Subsystem2/18(Out18) -> Bus Creator2/2
  Subsystem2/19(Out19) -> Bus Creator2/3
  Bus Creator2/1 -> [windshieldInputBus]
  Bus Selector/6 -> Subsystem/12(In13)  "<BRL_LED>"
  Bus Selector/2 -> Subsystem/8(In2)  "<GenericLedLinks>"
  Bus Selector/3 -> Subsystem/9(In3)  "<GenericLedRechts>"
  Bus Selector/4 -> Subsystem/10(In11)  "<GenericLedOben>"
  Bus Selector1/6 -> Subsystem/6(In10)  "<SchliessZustand>"
  Bus Selector1/1 -> Subsystem/1(In4)  "<down>"
  Bus Selector/5 -> Subsystem/11(In12)  "<RL_LED>"
  Bus Selector/8 -> Subsystem/14(In15)  "<NSL_LED>"
  Bus Selector/9 -> Subsystem/15(In16)  "<NSR_LED>"
  Bus Selector/13 -> Subsystem/19(In20)  "<RFL_LED>"
  [windshieldOutputBus] -> Bus Selector2/1
  Bus Selector2/1 -> Subsystem/21(In22)  "<down>"
  Bus Selector2/2 -> Subsystem/22(In23)  "<left>"
  Bus Selector2/3 -> Subsystem/23(In24)  "<right>"
  Bus Selector2/4 -> Subsystem/24(In25)  "<up>"
  Bus Selector2/5 -> Subsystem/25(In26)  "<SH_LED>"
  Bus Selector2/6 -> Subsystem/26(In27)  "<WW_LED>"
  Bus Selector2/7 -> Subsystem/27(In28)  "<SM_A>"
  Bus Selector2/8 -> Subsystem/28(In29)  "<SM_B>"
  Bus Selector2/9 -> Subsystem/29(In30)  "<SM_C>"
  Bus Selector2/10 -> Subsystem/30(In31)  "<SM_D>"
  Subsystem2/4(Out3) -> Bus Creator3/1
  Subsystem2/5(Out5) -> Bus Creator3/2
  Subsystem2/6(Out6) -> Bus Creator3/3
  Subsystem2/7(Out7) -> Bus Creator3/4
  Subsystem2/8(Out8) -> Bus Creator3/5
  Subsystem2/9(Out9) -> Bus Creator3/6
  Subsystem2/10(Out10) -> Bus Creator3/7
  Subsystem2/11(Out11) -> Bus Creator3/8
  Subsystem2/12(Out12) -> Bus Creator3/9
  Subsystem2/13(Out13) -> Bus Creator3/10
  Subsystem2/14(Out14) -> Bus Creator3/11
  Subsystem2/15(Out15) -> Bus Creator3/12
  Bus Creator3/1 -> [cockpitInputBus]
  Bus Selector9/3 -> Display_CanMsg_Cockpit_7/1  "<cockpitSteeringAngleDeg>"
  [cockpitInputBus] -> Bus Selector9/1
  Bus Selector9/1 -> Display_CanMsg_Cockpit_5/1  "<cockpitTemperature>"
  Bus Selector9/2 -> Display_CanMsg_Cockpit_6/1  "<cockpitVelocity>"

== system MBE_Simulation_04_Template_14_11_final/SchlossAlarmBox ==
  CanBus_SA_In : Inport
  SA_Box_Applikation : Subsystem
  SA_Box_Simulation_Input : Subsystem
  SA_Box_Simulation_Output : Subsystem
  CanBus_SA_Out : Outport
  wires:
  CanBus_SA_In/1 -> SA_Box_Simulation_Input/1(CanBus_SA_In)
  SA_Box_Simulation_Output/1(CanBus_SA_Out) -> CanBus_SA_Out/1
  SA_Box_Simulation_Input/7(CanTrigger_Bremse_2_Out) -> SA_Box_Applikation/7(CanTrigger_Bremse_2_In)
  SA_Box_Simulation_Input/6(CanData_Bremse_2_Out) -> SA_Box_Applikation/6(CanData_Bremse_2_In)
  SA_Box_Simulation_Input/5(CanTrigger_Cockpit_3_Out) -> SA_Box_Applikation/5(CanTrigger_Cockpit_3_In)
  SA_Box_Simulation_Input/4(CanData_Cockpit_3_Out) -> SA_Box_Applikation/4(CanData_Cockpit_3_In)
  SA_Box_Simulation_Input/3(AlarmButton_Out) -> SA_Box_Applikation/3(AlarmButton_In)
  SA_Box_Simulation_Input/2(SchliessButton_Out) -> SA_Box_Applikation/2(SchliessButton_In)
  SA_Box_Applikation/5(SchliessZustand_Out) -> SA_Box_Simulation_Output/5(SchliessZustand_LED_In)
  SA_Box_Applikation/6(AlarmZustand_Out) -> SA_Box_Simulation_Output/6(AlarmZustand_LED_In)
  SA_Box_Applikation/7(CanData_Alarm_1_Out) -> SA_Box_Simulation_Output/7(CanData_Alarm_1_In)
  SA_Box_Applikation/8(CanTrigger_Alarm_1_Out) -> SA_Box_Simulation_Output/8(CanTrigger_Alarm_1_In)
  SA_Box_Applikation/9(CanData_Schloss_1_Out) -> SA_Box_Simulation_Output/9(CanData_Schloss_1_In)
  SA_Box_Applikation/10(CanTrigger_Schloss_1_Out) -> SA_Box_Simulation_Output/10(CanTrigger_Schloss_1_In)
  SA_Box_Simulation_Input/1(GenericButton_Out) -> SA_Box_Applikation/1(GenericButton_In)
  SA_Box_Applikation/4(GenericLedOben_Out) -> SA_Box_Simulation_Output/4(GenericLedOben_LED_In)
  SA_Box_Applikation/3(GenericLedRechts_Out) -> SA_Box_Simulation_Output/3(GenericLedRechts_LED_In)
  SA_Box_Applikation/2(GenericLedLinks_Out) -> SA_Box_Simulation_Output/2(GenericLedLinks_LED_In)
  SA_Box_Applikation/1(GenericLedUnten_Out) -> SA_Box_Simulation_Output/1(GenericLedUnten_LED_In)

== system MBE_Simulation_04_Template_14_11_final/Slider Switch ==

== system MBE_Simulation_04_Template_14_11_final/WischerSensorBox ==
  CanBus_WS_In : Inport
  WS_Box_Applikation : Subsystem
  WS_Box_Simulation_Input : Subsystem
  WS_Box_Simulation_Output : Subsystem
  CanBus_WS_Out : Outport
  wires:
  CanBus_WS_In/1 -> WS_Box_Simulation_Input/1(CanBus_WS_In)
  WS_Box_Simulation_Output/1(CanBus_WS_Out) -> CanBus_WS_Out/1
  WS_Box_Simulation_Input/2(Lichtsensor_Out) -> WS_Box_Applikation/2(Lichtsensor_In)
  WS_Box_Simulation_Input/3(Distanzsensor_Out) -> WS_Box_Applikation/3(Distanzsensor_In)
  WS_Box_Simulation_Input/4(CanData_Cockpit_2_Out) -> WS_Box_Applikation/4(CanData_Cockpit_2_In)
  WS_Box_Simulation_Input/5(CanTrigger_Cockpit_2_Out) -> WS_Box_Applikation/5(CanTrigger_Cockpit_2_In)
  WS_Box_Simulation_Input/6(CanData_Schloss_1_Out) -> WS_Box_Applikation/6(CanData_Schloss_1_In)
  WS_Box_Simulation_Input/7(CanTrigger_Schloss_1_Out) -> WS_Box_Applikation/7(CanTrigger_Schloss_1_In)
  WS_Box_Simulation_Input/8(CanData_Bremse_2_Out) -> WS_Box_Applikation/8(CanData_Bremse_2_In)
  WS_Box_Simulation_Input/9(CanTrigger_Bremse_2_Out) -> WS_Box_Applikation/9(CanTrigger_Bremse_2_In)
  WS_Box_Applikation/5(CanData_Sensor_1_Out) -> WS_Box_Simulation_Output/5(CanData_Sensor_1_In)
  WS_Box_Applikation/6(CanTrigger_Sensor_1_Out) -> WS_Box_Simulation_Output/6(CanTrigger_Sensor_1_In)
  WS_Box_Applikation/7(SM_A_Out) -> WS_Box_Simulation_Output/7(SM_A_In)
  WS_Box_Applikation/8(SM_B_Out) -> WS_Box_Simulation_Output/8(SM_B_In)
  WS_Box_Applikation/9(SM_C_Out) -> WS_Box_Simulation_Output/9(SM_C_In)
  WS_Box_Applikation/10(SM_D_Out) -> WS_Box_Simulation_Output/10(SM_D_In)
  WS_Box_Applikation/11(WW_LED_Out) -> WS_Box_Simulation_Output/11(WW_LED_In)
  WS_Box_Applikation/12(SH_LED_Out) -> WS_Box_Simulation_Output/12(SH_LED_In)
  WS_Box_Simulation_Input/1(GenericButton_Out) -> WS_Box_Applikation/1(GenericButton_In)
  WS_Box_Applikation/4(GenericLedOben_Out) -> WS_Box_Simulation_Output/4(GenericLedOben_LED_In)
  WS_Box_Applikation/2(GenericLedLinks_Out) -> WS_Box_Simulation_Output/2(GenericLedLinks_LED_In)
  WS_Box_Applikation/1(GenericLedUnten_Out) -> WS_Box_Simulation_Output/1(GenericLedUnten_LED_In)
  WS_Box_Applikation/3(GenericLedRechts_Out) -> WS_Box_Simulation_Output/3(GenericLedRechts_LED_In)

== system MBE_Simulation_04_Template_14_11_final/Cockpit/CanBus_Cockpit ==
  "CanMsg_Cockpit_1_In " : Inport
  CanMsg_Cockpit_2_In : Inport  Port=2
  CanMsg_Cockpit_3_In : Inport  Port=3
  CanMsg_Cockpit_4_In : Inport  Port=4
  CanMsg_Bremse_1_In : Inport  Port=5
  CanMsg_Bremse_2_In : Inport  Port=6
  Bus Creator4 : BusCreator  Inputs=6
  CanBus_Cockpit_Out : Outport
  wires:
  CanMsg_Cockpit_3_In/1 -> Bus Creator4/3
  "CanMsg_Cockpit_1_In "/1 -> Bus Creator4/1
  CanMsg_Cockpit_4_In/1 -> Bus Creator4/4
  CanMsg_Bremse_2_In/1 -> Bus Creator4/6
  CanMsg_Cockpit_2_In/1 -> Bus Creator4/2
  Bus Creator4/1 -> CanBus_Cockpit_Out/1  "CanBus_Cockpit"
  CanMsg_Bremse_1_In/1 -> Bus Creator4/5

== system MBE_Simulation_04_Template_14_11_final/Cockpit/CanCoder_Bremse_1 ==
  Bremse_In : Inport
  Warnbremsung_In : Inport  Port=2
  Notbremsungl_In : Inport  Port=3
  Bitwise Operator3 : simulink/Logic and Bit Operations/Bitwise Operator  logicop=OR  UseBitMask=off  NumInputPorts=3  BitMask=bin2dec('11011001')  BitMaskRealWorld=Stored Integer
  Gain4 : Gain  Gain=2^0  OutDataTypeStr=uint8
  Gain8 : Gain  Gain=2^1  OutDataTypeStr=uint8
  Gain9 : Gain  Gain=2^2  OutDataTypeStr=uint8
  TriggerPuls : Subsystem
  CanData_Bremse_1 : Outport
  CanTrigger_Bremse_1 : Outport  Port=2
  wires:
  Notbremsungl_In/1 -> Gain9/1
  Bremse_In/1 -> Gain4/1
  Gain9/1 -> Bitwise Operator3/3
  Gain4/1 -> Bitwise Operator3/1
  Gain8/1 -> Bitwise Operator3/2
  Bitwise Operator3/1 -> CanData_Bremse_1/1
  Warnbremsung_In/1 -> Gain8/1
  TriggerPuls/1(TriggerPuls_100ms) -> CanTrigger_Bremse_1/1

== system MBE_Simulation_04_Template_14_11_final/Cockpit/CanCoder_Bremse_2 ==
  GeschwindigkeitsSlider_In : Inport
  Detect Change4 : simulink/Logic and Bit Operations/Detect Change  vinit=0  OutDataTypeStr=boolean
  Gain : Gain  Gain=2^0  OutDataTypeStr=uint8
  CanMsg_Bremse_2 : Outport
  CanTrigger_Bremse_2 : Outport  Port=2
  wires:
  Gain/1 -> CanMsg_Bremse_2/1
  GeschwindigkeitsSlider_In/1 -> Detect Change4/1, Gain/1
  Detect Change4/1 -> CanTrigger_Bremse_2/1

== system MBE_Simulation_04_Template_14_11_final/Cockpit/CanCoder_Cockpit_1 ==
  Lichtschalter_In : Inport
  Blinkerhebel_In : Inport  Port=2
  Warnblinker : Inport  Port=3
  Bitwise Operator3 : simulink/Logic and Bit Operations/Bitwise Operator  logicop=OR  UseBitMask=off  NumInputPorts=3  BitMask=bin2dec('11011001')  BitMaskRealWorld=Stored Integer
  Bitwise Operator4 : simulink/Logic and Bit Operations/Bitwise Operator  logicop=OR  UseBitMask=off  NumInputPorts=2  BitMask=bin2dec('11011001')  BitMaskRealWorld=Stored Integer
  Data Type Conversion8 : DataTypeConversion  OutDataTypeStr=uint8
  Direct Lookup Table (n-D) : LookupNDDirect  NumberOfTableDimensions=1  Table=[2; 1; 0; 0; 0]
  Direct Lookup Table (n-D)1 : LookupNDDirect  NumberOfTableDimensions=1  Table=[0; 0; 0; 1; 2]
  Direct Lookup Table (n-D)2 : LookupNDDirect  NumberOfTableDimensions=1  Table=[1; 0; 2; 3; 4]
  Gain10 : Gain  Gain=2^5  OutDataTypeStr=uint8
  Gain4 : Gain  Gain=2^0  OutDataTypeStr=uint8
  Gain7 : Gain  Gain=2^7  OutDataTypeStr=uint8
  Gain9 : Gain  Gain=2^3  OutDataTypeStr=uint8
  TriggerPuls : Subsystem
  CanData_Cockpit_1 : Outport
  CanTrigger_Cockpit_1 : Outport  Port=2
  wires:
  Bitwise Operator3/1 -> CanData_Cockpit_1/1
  Gain7/1 -> Bitwise Operator3/3
  Data Type Conversion8/1 -> Gain7/1
  Gain4/1 -> Bitwise Operator3/1
  Direct Lookup Table (n-D)1/1 -> Gain9/1
  Direct Lookup Table (n-D)/1 -> Gain10/1
  Gain9/1 -> Bitwise Operator4/1
  Gain10/1 -> Bitwise Operator4/2
  Bitwise Operator4/1 -> Bitwise Operator3/2
  Direct Lookup Table (n-D)2/1 -> Gain4/1
  Warnblinker/1 -> Data Type Conversion8/1
  Lichtschalter_In/1 -> Direct Lookup Table (n-D)2/1
  Blinkerhebel_In/1 -> Direct Lookup Table (n-D)/1, Direct Lookup Table (n-D)1/1
  TriggerPuls/1(TriggerPuls_200ms) -> CanTrigger_Cockpit_1/1
